simulink model "Ecm_2RC_battery"  (R2022a)
settings: Solver=FixedStepAuto  StartTime=0.0  StopTime=3600  FixedStep=0.1  RelTol=1e-3
values from neighbouring files (symbols this model uses):
  T_init = 293.15    [cell_data.mat]
libraries: fl_lib x1074, LiBatteryElements_lib x540, nesl_utility x102
(part 16 of 18)

== system Ecm_2RC_battery/Subsystem3/Subsystem2/Thermal Model ==
  Battery Thermal Mass : fl_lib/Thermal/Thermal Elements/Thermal Mass  mass=cell_mass kg  sp_heat=cell_Cp_heat J/kg/K  T_specify=on  T_priority=High  T=T_init K  T_nominal_specify=off  T_nominal_unit=K  T_nominal_value=1  Q_specify=off  Q_priority=None  Q=0 W  Q_nominal_specify=off  Q_nominal_unit=W  Q_nominal_value=1
      settings: SourceProductBaseCode=PW,SS,VE
  Controlled Heat Flow Rate Source : fl_lib/Thermal/Thermal Sources/Controlled Heat Flow Rate Source
      settings: SourceProductBaseCode=PW,SS,VE
  Temperature Sensor : fl_lib/Thermal/Thermal Sensors/Temperature Sensor
      settings: SourceProductBaseCode=PW,SS,VE
  Thermal Reference : fl_lib/Thermal/Thermal Elements/Thermal Reference
      settings: SourceProductBaseCode=PW,SS,VE
  Thermal Reference1 : fl_lib/Thermal/Thermal Elements/Thermal Reference
      settings: SourceProductBaseCode=PW,SS,VE
  P_in : PMIOPort  Tag=PMCPort  Side=Left
  H : PMIOPort  Tag=PMCPort  Port=2  Side=Left
  T : PMIOPort  Tag=PMCPort  Port=3  Side=Right
  connections:
  Temperature Sensor/RConn1 -- Thermal Reference1/LConn1
  Temperature Sensor/RConn2 -- T/RConn1
  Controlled Heat Flow Rate Source/RConn2 -- Thermal Reference/LConn1
  Controlled Heat Flow Rate Source/LConn1 -- Temperature Sensor/LConn1 -- Battery Thermal Mass/LConn1 -- H/RConn1
  Controlled Heat Flow Rate Source/RConn1 -- P_in/RConn1

== system Ecm_2RC_battery/Subsystem3/Subsystem3/Sum ==
  Power Sum : fl_lib/Physical Signals/Functions/PS Add
      settings: SourceProductBaseCode=PW,SS,VE
  Power Sum1 : fl_lib/Physical Signals/Functions/PS Add
      settings: SourceProductBaseCode=PW,SS,VE
  I1 : PMIOPort  Side=Right
  I2 : PMIOPort  Port=2  Side=Right
  I3 : PMIOPort  Port=3  Side=Right
  O : PMIOPort  Port=4  Side=Left
  connections:
  Power Sum1/LConn1 -- I2/RConn1
  Power Sum/RConn1 -- O/RConn1
  I3/RConn1 -- Power Sum1/LConn2
  Power Sum1/RConn1 -- Power Sum/LConn2
  I1/RConn1 -- Power Sum/LConn1

== system Ecm_2RC_battery/Subsystem3/Subsystem3/Thermal Model ==
  Battery Thermal Mass : fl_lib/Thermal/Thermal Elements/Thermal Mass  mass=cell_mass kg  sp_heat=cell_Cp_heat J/kg/K  T_specify=on  T_priority=High  T=T_init K  T_nominal_specify=off  T_nominal_unit=K  T_nominal_value=1  Q_specify=off  Q_priority=None  Q=0 W  Q_nominal_specify=off  Q_nominal_unit=W  Q_nominal_value=1
      settings: SourceProductBaseCode=PW,SS,VE
  Controlled Heat Flow Rate Source : fl_lib/Thermal/Thermal Sources/Controlled Heat Flow Rate Source
      settings: SourceProductBaseCode=PW,SS,VE
  Temperature Sensor : fl_lib/Thermal/Thermal Sensors/Temperature Sensor
      settings: SourceProductBaseCode=PW,SS,VE
  Thermal Reference : fl_lib/Thermal/Thermal Elements/Thermal Reference
      settings: SourceProductBaseCode=PW,SS,VE
  Thermal Reference1 : fl_lib/Thermal/Thermal Elements/Thermal Reference
      settings: SourceProductBaseCode=PW,SS,VE
  P_in : PMIOPort  Tag=PMCPort  Side=Left
  H : PMIOPort  Tag=PMCPort  Port=2  Side=Left
  T : PMIOPort  Tag=PMCPort  Port=3  Side=Right
  connections:
  Temperature Sensor/RConn1 -- Thermal Reference1/LConn1
  Temperature Sensor/RConn2 -- T/RConn1
  Controlled Heat Flow Rate Source/RConn2 -- Thermal Reference/LConn1
  Controlled Heat Flow Rate Source/LConn1 -- Temperature Sensor/LConn1 -- Battery Thermal Mass/LConn1 -- H/RConn1
  Controlled Heat Flow Rate Source/RConn1 -- P_in/RConn1

== system Ecm_2RC_battery/Subsystem3/Subsystem4/Sum ==
  Power Sum : fl_lib/Physical Signals/Functions/PS Add
      settings: SourceProductBaseCode=PW,SS,VE
  Power Sum1 : fl_lib/Physical Signals/Functions/PS Add
      settings: SourceProductBaseCode=PW,SS,VE
  I1 : PMIOPort  Side=Right
  I2 : PMIOPort  Port=2  Side=Right
  I3 : PMIOPort  Port=3  Side=Right
  O : PMIOPort  Port=4  Side=Left
  connections:
  Power Sum1/LConn1 -- I2/RConn1
  Power Sum/RConn1 -- O/RConn1
  I3/RConn1 -- Power Sum1/LConn2
  Power Sum1/RConn1 -- Power Sum/LConn2
  I1/RConn1 -- Power Sum/LConn1

== system Ecm_2RC_battery/Subsystem3/Subsystem4/Thermal Model ==
  Battery Thermal Mass : fl_lib/Thermal/Thermal Elements/Thermal Mass  mass=cell_mass kg  sp_heat=cell_Cp_heat J/kg/K  T_specify=on  T_priority=High  T=T_init K  T_nominal_specify=off  T_nominal_unit=K  T_nominal_value=1  Q_specify=off  Q_priority=None  Q=0 W  Q_nominal_specify=off  Q_nominal_unit=W  Q_nominal_value=1
      settings: SourceProductBaseCode=PW,SS,VE
  Controlled Heat Flow Rate Source : fl_lib/Thermal/Thermal Sources/Controlled Heat Flow Rate Source
      settings: SourceProductBaseCode=PW,SS,VE
  Temperature Sensor : fl_lib/Thermal/Thermal Sensors/Temperature Sensor
      settings: SourceProductBaseCode=PW,SS,VE
  Thermal Reference : fl_lib/Thermal/Thermal Elements/Thermal Reference
      settings: SourceProductBaseCode=PW,SS,VE
  Thermal Reference1 : fl_lib/Thermal/Thermal Elements/Thermal Reference
      settings: SourceProductBaseCode=PW,SS,VE
  P_in : PMIOPort  Tag=PMCPort  Side=Left
  H : PMIOPort  Tag=PMCPort  Port=2  Side=Left
  T : PMIOPort  Tag=PMCPort  Port=3  Side=Right
  connections:
  Temperature Sensor/RConn1 -- Thermal Reference1/LConn1
  Temperature Sensor/RConn2 -- T/RConn1
  Controlled Heat Flow Rate Source/RConn2 -- Thermal Reference/LConn1
  Controlled Heat Flow Rate Source/LConn1 -- Temperature Sensor/LConn1 -- Battery Thermal Mass/LConn1 -- H/RConn1
  Controlled Heat Flow Rate Source/RConn1 -- P_in/RConn1

== system Ecm_2RC_battery/Subsystem3/Subsystem5/Sum ==
  Power Sum : fl_lib/Physical Signals/Functions/PS Add
      settings: SourceProductBaseCode=PW,SS,VE
  Power Sum1 : fl_lib/Physical Signals/Functions/PS Add
      settings: SourceProductBaseCode=PW,SS,VE
  I1 : PMIOPort  Side=Right
  I2 : PMIOPort  Port=2  Side=Right
  I3 : PMIOPort  Port=3  Side=Right
  O : PMIOPort  Port=4  Side=Left
  connections:
  Power Sum1/LConn1 -- I2/RConn1
  Power Sum/RConn1 -- O/RConn1
  I3/RConn1 -- Power Sum1/LConn2
  Power Sum1/RConn1 -- Power Sum/LConn2
  I1/RConn1 -- Power Sum/LConn1

== system Ecm_2RC_battery/Subsystem3/Subsystem5/Thermal Model ==
  Battery Thermal Mass : fl_lib/Thermal/Thermal Elements/Thermal Mass  mass=cell_mass kg  sp_heat=cell_Cp_heat J/kg/K  T_specify=on  T_priority=High  T=T_init K  T_nominal_specify=off  T_nominal_unit=K  T_nominal_value=1  Q_specify=off  Q_priority=None  Q=0 W  Q_nominal_specify=off  Q_nominal_unit=W  Q_nominal_value=1
      settings: SourceProductBaseCode=PW,SS,VE
  Controlled Heat Flow Rate Source : fl_lib/Thermal/Thermal Sources/Controlled Heat Flow Rate Source
      settings: SourceProductBaseCode=PW,SS,VE
  Temperature Sensor : fl_lib/Thermal/Thermal Sensors/Temperature Sensor
      settings: SourceProductBaseCode=PW,SS,VE
  Thermal Reference : fl_lib/Thermal/Thermal Elements/Thermal Reference
      settings: SourceProductBaseCode=PW,SS,VE
  Thermal Reference1 : fl_lib/Thermal/Thermal Elements/Thermal Reference
      settings: SourceProductBaseCode=PW,SS,VE
  P_in : PMIOPort  Tag=PMCPort  Side=Left
  H : PMIOPort  Tag=PMCPort  Port=2  Side=Left
  T : PMIOPort  Tag=PMCPort  Port=3  Side=Right
  connections:
  Temperature Sensor/RConn1 -- Thermal Reference1/LConn1
  Temperature Sensor/RConn2 -- T/RConn1
  Controlled Heat Flow Rate Source/RConn2 -- Thermal Reference/LConn1
  Controlled Heat Flow Rate Source/LConn1 -- Temperature Sensor/LConn1 -- Battery Thermal Mass/LConn1 -- H/RConn1
  Controlled Heat Flow Rate Source/RConn1 -- P_in/RConn1

== system Ecm_2RC_battery/Subsystem3/Subsystem6/Sum ==
  Power Sum : fl_lib/Physical Signals/Functions/PS Add
      settings: SourceProductBaseCode=PW,SS,VE
  Power Sum1 : fl_lib/Physical Signals/Functions/PS Add
      settings: SourceProductBaseCode=PW,SS,VE
  I1 : PMIOPort  Side=Right
  I2 : PMIOPort  Port=2  Side=Right
  I3 : PMIOPort  Port=3  Side=Right
  O : PMIOPort  Port=4  Side=Left
  connections:
  Power Sum1/LConn1 -- I2/RConn1
  Power Sum/RConn1 -- O/RConn1
  I3/RConn1 -- Power Sum1/LConn2
  Power Sum1/RConn1 -- Power Sum/LConn2
  I1/RConn1 -- Power Sum/LConn1

== system Ecm_2RC_battery/Subsystem3/Subsystem6/Thermal Model ==
  Battery Thermal Mass : fl_lib/Thermal/Thermal Elements/Thermal Mass  mass=cell_mass kg  sp_heat=cell_Cp_heat J/kg/K  T_specify=on  T_priority=High  T=T_init K  T_nominal_specify=off  T_nominal_unit=K  T_nominal_value=1  Q_specify=off  Q_priority=None  Q=0 W  Q_nominal_specify=off  Q_nominal_unit=W  Q_nominal_value=1
      settings: SourceProductBaseCode=PW,SS,VE
  Controlled Heat Flow Rate Source : fl_lib/Thermal/Thermal Sources/Controlled Heat Flow Rate Source
      settings: SourceProductBaseCode=PW,SS,VE
  Temperature Sensor : fl_lib/Thermal/Thermal Sensors/Temperature Sensor
      settings: SourceProductBaseCode=PW,SS,VE
  Thermal Reference : fl_lib/Thermal/Thermal Elements/Thermal Reference
      settings: SourceProductBaseCode=PW,SS,VE
  Thermal Reference1 : fl_lib/Thermal/Thermal Elements/Thermal Reference
      settings: SourceProductBaseCode=PW,SS,VE
  P_in : PMIOPort  Tag=PMCPort  Side=Left
  H : PMIOPort  Tag=PMCPort  Port=2  Side=Left
  T : PMIOPort  Tag=PMCPort  Port=3  Side=Right
  connections:
  Temperature Sensor/RConn1 -- Thermal Reference1/LConn1
  Temperature Sensor/RConn2 -- T/RConn1
  Controlled Heat Flow Rate Source/RConn2 -- Thermal Reference/LConn1
  Controlled Heat Flow Rate Source/LConn1 -- Temperature Sensor/LConn1 -- Battery Thermal Mass/LConn1 -- H/RConn1
  Controlled Heat Flow Rate Source/RConn1 -- P_in/RConn1

== system Ecm_2RC_battery/Subsystem3/Subsystem7/Sum ==
  Power Sum : fl_lib/Physical Signals/Functions/PS Add
      settings: SourceProductBaseCode=PW,SS,VE
  Power Sum1 : fl_lib/Physical Signals/Functions/PS Add
      settings: SourceProductBaseCode=PW,SS,VE
  I1 : PMIOPort  Side=Right
  I2 : PMIOPort  Port=2  Side=Right
  I3 : PMIOPort  Port=3  Side=Right
  O : PMIOPort  Port=4  Side=Left
  connections:
  Power Sum1/LConn1 -- I2/RConn1
  Power Sum/RConn1 -- O/RConn1
  I3/RConn1 -- Power Sum1/LConn2
  Power Sum1/RConn1 -- Power Sum/LConn2
  I1/RConn1 -- Power Sum/LConn1

== system Ecm_2RC_battery/Subsystem3/Subsystem7/Thermal Model ==
  Battery Thermal Mass : fl_lib/Thermal/Thermal Elements/Thermal Mass  mass=cell_mass kg  sp_heat=cell_Cp_heat J/kg/K  T_specify=on  T_priority=High  T=T_init K  T_nominal_specify=off  T_nominal_unit=K  T_nominal_value=1  Q_specify=off  Q_priority=None  Q=0 W  Q_nominal_specify=off  Q_nominal_unit=W  Q_nominal_value=1
      settings: SourceProductBaseCode=PW,SS,VE
  Controlled Heat Flow Rate Source : fl_lib/Thermal/Thermal Sources/Controlled Heat Flow Rate Source
      settings: SourceProductBaseCode=PW,SS,VE
  Temperature Sensor : fl_lib/Thermal/Thermal Sensors/Temperature Sensor
      settings: SourceProductBaseCode=PW,SS,VE
  Thermal Reference : fl_lib/Thermal/Thermal Elements/Thermal Reference
      settings: SourceProductBaseCode=PW,SS,VE
  Thermal Reference1 : fl_lib/Thermal/Thermal Elements/Thermal Reference
      settings: SourceProductBaseCode=PW,SS,VE
  P_in : PMIOPort  Tag=PMCPort  Side=Left
  H : PMIOPort  Tag=PMCPort  Port=2  Side=Left
  T : PMIOPort  Tag=PMCPort  Port=3  Side=Right
  connections:
  Temperature Sensor/RConn1 -- Thermal Reference1/LConn1
  Temperature Sensor/RConn2 -- T/RConn1
  Controlled Heat Flow Rate Source/RConn2 -- Thermal Reference/LConn1
  Controlled Heat Flow Rate Source/LConn1 -- Temperature Sensor/LConn1 -- Battery Thermal Mass/LConn1 -- H/RConn1
  Controlled Heat Flow Rate Source/RConn1 -- P_in/RConn1

== system Ecm_2RC_battery/Subsystem3/Subsystem8/Sum ==
  Power Sum : fl_lib/Physical Signals/Functions/PS Add
      settings: SourceProductBaseCode=PW,SS,VE
  Power Sum1 : fl_lib/Physical Signals/Functions/PS Add
      settings: SourceProductBaseCode=PW,SS,VE
  I1 : PMIOPort  Side=Right
  I2 : PMIOPort  Port=2  Side=Right
  I3 : PMIOPort  Port=3  Side=Right
  O : PMIOPort  Port=4  Side=Left
  connections:
  Power Sum1/LConn1 -- I2/RConn1
  Power Sum/RConn1 -- O/RConn1
  I3/RConn1 -- Power Sum1/LConn2
  Power Sum1/RConn1 -- Power Sum/LConn2
  I1/RConn1 -- Power Sum/LConn1

== system Ecm_2RC_battery/Subsystem3/Subsystem8/Thermal Model ==
  Battery Thermal Mass : fl_lib/Thermal/Thermal Elements/Thermal Mass  mass=cell_mass kg  sp_heat=cell_Cp_heat J/kg/K  T_specify=on  T_priority=High  T=T_init K  T_nominal_specify=off  T_nominal_unit=K  T_nominal_value=1  Q_specify=off  Q_priority=None  Q=0 W  Q_nominal_specify=off  Q_nominal_unit=W  Q_nominal_value=1
      settings: SourceProductBaseCode=PW,SS,VE
  Controlled Heat Flow Rate Source : fl_lib/Thermal/Thermal Sources/Controlled Heat Flow Rate Source
      settings: SourceProductBaseCode=PW,SS,VE
  Temperature Sensor : fl_lib/Thermal/Thermal Sensors/Temperature Sensor
      settings: SourceProductBaseCode=PW,SS,VE
  Thermal Reference : fl_lib/Thermal/Thermal Elements/Thermal Reference
      settings: SourceProductBaseCode=PW,SS,VE
  Thermal Reference1 : fl_lib/Thermal/Thermal Elements/Thermal Reference
      settings: SourceProductBaseCode=PW,SS,VE
  P_in : PMIOPort  Tag=PMCPort  Side=Left
  H : PMIOPort  Tag=PMCPort  Port=2  Side=Left
  T : PMIOPort  Tag=PMCPort  Port=3  Side=Right
  connections:
  Temperature Sensor/RConn1 -- Thermal Reference1/LConn1
  Temperature Sensor/RConn2 -- T/RConn1
  Controlled Heat Flow Rate Source/RConn2 -- Thermal Reference/LConn1
  Controlled Heat Flow Rate Source/LConn1 -- Temperature Sensor/LConn1 -- Battery Thermal Mass/LConn1 -- H/RConn1
  Controlled Heat Flow Rate Source/RConn1 -- P_in/RConn1

== system Ecm_2RC_battery/Subsystem3/Subsystem9/Sum ==
  Power Sum : fl_lib/Physical Signals/Functions/PS Add
      settings: SourceProductBaseCode=PW,SS,VE
  Power Sum1 : fl_lib/Physical Signals/Functions/PS Add
      settings: SourceProductBaseCode=PW,SS,VE
  I1 : PMIOPort  Side=Right
  I2 : PMIOPort  Port=2  Side=Right
  I3 : PMIOPort  Port=3  Side=Right
  O : PMIOPort  Port=4  Side=Left
  connections:
  Power Sum1/LConn1 -- I2/RConn1
  Power Sum/RConn1 -- O/RConn1
  I3/RConn1 -- Power Sum1/LConn2
  Power Sum1/RConn1 -- Power Sum/LConn2
  I1/RConn1 -- Power Sum/LConn1

== system Ecm_2RC_battery/Subsystem3/Subsystem9/Thermal Model ==
  Battery Thermal Mass : fl_lib/Thermal/Thermal Elements/Thermal Mass  mass=cell_mass kg  sp_heat=cell_Cp_heat J/kg/K  T_specify=on  T_priority=High  T=T_init K  T_nominal_specify=off  T_nominal_unit=K  T_nominal_value=1  Q_specify=off  Q_priority=None  Q=0 W  Q_nominal_specify=off  Q_nominal_unit=W  Q_nominal_value=1
      settings: SourceProductBaseCode=PW,SS,VE
  Controlled Heat Flow Rate Source : fl_lib/Thermal/Thermal Sources/Controlled Heat Flow Rate Source
      settings: SourceProductBaseCode=PW,SS,VE
  Temperature Sensor : fl_lib/Thermal/Thermal Sensors/Temperature Sensor
      settings: SourceProductBaseCode=PW,SS,VE
  Thermal Reference : fl_lib/Thermal/Thermal Elements/Thermal Reference
      settings: SourceProductBaseCode=PW,SS,VE
  Thermal Reference1 : fl_lib/Thermal/Thermal Elements/Thermal Reference
      settings: SourceProductBaseCode=PW,SS,VE
  P_in : PMIOPort  Tag=PMCPort  Side=Left
  H : PMIOPort  Tag=PMCPort  Port=2  Side=Left
  T : PMIOPort  Tag=PMCPort  Port=3  Side=Right
  connections:
  Temperature Sensor/RConn1 -- Thermal Reference1/LConn1
  Temperature Sensor/RConn2 -- T/RConn1
  Controlled Heat Flow Rate Source/RConn2 -- Thermal Reference/LConn1
  Controlled Heat Flow Rate Source/LConn1 -- Temperature Sensor/LConn1 -- Battery Thermal Mass/LConn1 -- H/RConn1
  Controlled Heat Flow Rate Source/RConn1 -- P_in/RConn1

== system Ecm_2RC_battery/Subsystem4/Subsystem/Sum ==
  Power Sum : fl_lib/Physical Signals/Functions/PS Add
      settings: SourceProductBaseCode=PW,SS,VE
  Power Sum1 : fl_lib/Physical Signals/Functions/PS Add
      settings: SourceProductBaseCode=PW,SS,VE
  I1 : PMIOPort  Side=Right
  I2 : PMIOPort  Port=2  Side=Right
  I3 : PMIOPort  Port=3  Side=Right
  O : PMIOPort  Port=4  Side=Left
  connections:
  Power Sum1/LConn1 -- I2/RConn1
  Power Sum/RConn1 -- O/RConn1
  I3/RConn1 -- Power Sum1/LConn2
  Power Sum1/RConn1 -- Power Sum/LConn2
  I1/RConn1 -- Power Sum/LConn1

== system Ecm_2RC_battery/Subsystem4/Subsystem/Thermal Model ==
  Battery Thermal Mass : fl_lib/Thermal/Thermal Elements/Thermal Mass  mass=cell_mass kg  sp_heat=cell_Cp_heat J/kg/K  T_specify=on  T_priority=High  T=T_init K  T_nominal_specify=off  T_nominal_unit=K  T_nominal_value=1  Q_specify=off  Q_priority=None  Q=0 W  Q_nominal_specify=off  Q_nominal_unit=W  Q_nominal_value=1
      settings: SourceProductBaseCode=PW,SS,VE
  Controlled Heat Flow Rate Source : fl_lib/Thermal/Thermal Sources/Controlled Heat Flow Rate Source
      settings: SourceProductBaseCode=PW,SS,VE
  Temperature Sensor : fl_lib/Thermal/Thermal Sensors/Temperature Sensor
      settings: SourceProductBaseCode=PW,SS,VE
  Thermal Reference : fl_lib/Thermal/Thermal Elements/Thermal Reference
      settings: SourceProductBaseCode=PW,SS,VE
  Thermal Reference1 : fl_lib/Thermal/Thermal Elements/Thermal Reference
      settings: SourceProductBaseCode=PW,SS,VE
  P_in : PMIOPort  Tag=PMCPort  Side=Left
  H : PMIOPort  Tag=PMCPort  Port=2  Side=Left
  T : PMIOPort  Tag=PMCPort  Port=3  Side=Right
  connections:
  Temperature Sensor/RConn1 -- Thermal Reference1/LConn1
  Temperature Sensor/RConn2 -- T/RConn1
  Controlled Heat Flow Rate Source/RConn2 -- Thermal Reference/LConn1
  Controlled Heat Flow Rate Source/LConn1 -- Temperature Sensor/LConn1 -- Battery Thermal Mass/LConn1 -- H/RConn1
  Controlled Heat Flow Rate Source/RConn1 -- P_in/RConn1

== system Ecm_2RC_battery/Subsystem4/Subsystem1/Sum ==
  Power Sum : fl_lib/Physical Signals/Functions/PS Add
      settings: SourceProductBaseCode=PW,SS,VE
  Power Sum1 : fl_lib/Physical Signals/Functions/PS Add
      settings: SourceProductBaseCode=PW,SS,VE
  I1 : PMIOPort  Side=Right
  I2 : PMIOPort  Port=2  Side=Right
  I3 : PMIOPort  Port=3  Side=Right
  O : PMIOPort  Port=4  Side=Left
  connections:
  Power Sum1/LConn1 -- I2/RConn1
  Power Sum/RConn1 -- O/RConn1
  I3/RConn1 -- Power Sum1/LConn2
  Power Sum1/RConn1 -- Power Sum/LConn2
  I1/RConn1 -- Power Sum/LConn1

== system Ecm_2RC_battery/Subsystem4/Subsystem1/Thermal Model ==
  Battery Thermal Mass : fl_lib/Thermal/Thermal Elements/Thermal Mass  mass=cell_mass kg  sp_heat=cell_Cp_heat J/kg/K  T_specify=on  T_priority=High  T=T_init K  T_nominal_specify=off  T_nominal_unit=K  T_nominal_value=1  Q_specify=off  Q_priority=None  Q=0 W  Q_nominal_specify=off  Q_nominal_unit=W  Q_nominal_value=1
      settings: SourceProductBaseCode=PW,SS,VE
  Controlled Heat Flow Rate Source : fl_lib/Thermal/Thermal Sources/Controlled Heat Flow Rate Source
      settings: SourceProductBaseCode=PW,SS,VE
  Temperature Sensor : fl_lib/Thermal/Thermal Sensors/Temperature Sensor
      settings: SourceProductBaseCode=PW,SS,VE
  Thermal Reference : fl_lib/Thermal/Thermal Elements/Thermal Reference
      settings: SourceProductBaseCode=PW,SS,VE
  Thermal Reference1 : fl_lib/Thermal/Thermal Elements/Thermal Reference
      settings: SourceProductBaseCode=PW,SS,VE
  P_in : PMIOPort  Tag=PMCPort  Side=Left
  H : PMIOPort  Tag=PMCPort  Port=2  Side=Left
  T : PMIOPort  Tag=PMCPort  Port=3  Side=Right
  connections:
  Temperature Sensor/RConn1 -- Thermal Reference1/LConn1
  Temperature Sensor/RConn2 -- T/RConn1
  Controlled Heat Flow Rate Source/RConn2 -- Thermal Reference/LConn1
  Controlled Heat Flow Rate Source/LConn1 -- Temperature Sensor/LConn1 -- Battery Thermal Mass/LConn1 -- H/RConn1
  Controlled Heat Flow Rate Source/RConn1 -- P_in/RConn1

== system Ecm_2RC_battery/Subsystem4/Subsystem2/Sum ==
  Power Sum : fl_lib/Physical Signals/Functions/PS Add
      settings: SourceProductBaseCode=PW,SS,VE
  Power Sum1 : fl_lib/Physical Signals/Functions/PS Add
      settings: SourceProductBaseCode=PW,SS,VE
  I1 : PMIOPort  Side=Right
  I2 : PMIOPort  Port=2  Side=Right
  I3 : PMIOPort  Port=3  Side=Right
  O : PMIOPort  Port=4  Side=Left
  connections:
  Power Sum1/LConn1 -- I2/RConn1
  Power Sum/RConn1 -- O/RConn1
  I3/RConn1 -- Power Sum1/LConn2
  Power Sum1/RConn1 -- Power Sum/LConn2
  I1/RConn1 -- Power Sum/LConn1

== system Ecm_2RC_battery/Subsystem4/Subsystem2/Thermal Model ==
  Battery Thermal Mass : fl_lib/Thermal/Thermal Elements/Thermal Mass  mass=cell_mass kg  sp_heat=cell_Cp_heat J/kg/K  T_specify=on  T_priority=High  T=T_init K  T_nominal_specify=off  T_nominal_unit=K  T_nominal_value=1  Q_specify=off  Q_priority=None  Q=0 W  Q_nominal_specify=off  Q_nominal_unit=W  Q_nominal_value=1
      settings: SourceProductBaseCode=PW,SS,VE
  Controlled Heat Flow Rate Source : fl_lib/Thermal/Thermal Sources/Controlled Heat Flow Rate Source
      settings: SourceProductBaseCode=PW,SS,VE
  Temperature Sensor : fl_lib/Thermal/Thermal Sensors/Temperature Sensor
      settings: SourceProductBaseCode=PW,SS,VE
  Thermal Reference : fl_lib/Thermal/Thermal Elements/Thermal Reference
      settings: SourceProductBaseCode=PW,SS,VE
  Thermal Reference1 : fl_lib/Thermal/Thermal Elements/Thermal Reference
      settings: SourceProductBaseCode=PW,SS,VE
  P_in : PMIOPort  Tag=PMCPort  Side=Left
  H : PMIOPort  Tag=PMCPort  Port=2  Side=Left
  T : PMIOPort  Tag=PMCPort  Port=3  Side=Right
  connections:
  Temperature Sensor/RConn1 -- Thermal Reference1/LConn1
  Temperature Sensor/RConn2 -- T/RConn1
  Controlled Heat Flow Rate Source/RConn2 -- Thermal Reference/LConn1
  Controlled Heat Flow Rate Source/LConn1 -- Temperature Sensor/LConn1 -- Battery Thermal Mass/LConn1 -- H/RConn1
  Controlled Heat Flow Rate Source/RConn1 -- P_in/RConn1

== system Ecm_2RC_battery/Subsystem4/Subsystem3/Sum ==
  Power Sum : fl_lib/Physical Signals/Functions/PS Add
      settings: SourceProductBaseCode=PW,SS,VE
  Power Sum1 : fl_lib/Physical Signals/Functions/PS Add
      settings: SourceProductBaseCode=PW,SS,VE
  I1 : PMIOPort  Side=Right
  I2 : PMIOPort  Port=2  Side=Right
  I3 : PMIOPort  Port=3  Side=Right
  O : PMIOPort  Port=4  Side=Left
  connections:
  Power Sum1/LConn1 -- I2/RConn1
  Power Sum/RConn1 -- O/RConn1
  I3/RConn1 -- Power Sum1/LConn2
  Power Sum1/RConn1 -- Power Sum/LConn2
  I1/RConn1 -- Power Sum/LConn1

== system Ecm_2RC_battery/Subsystem4/Subsystem3/Thermal Model ==
  Battery Thermal Mass : fl_lib/Thermal/Thermal Elements/Thermal Mass  mass=cell_mass kg  sp_heat=cell_Cp_heat J/kg/K  T_specify=on  T_priority=High  T=T_init K  T_nominal_specify=off  T_nominal_unit=K  T_nominal_value=1  Q_specify=off  Q_priority=None  Q=0 W  Q_nominal_specify=off  Q_nominal_unit=W  Q_nominal_value=1
      settings: SourceProductBaseCode=PW,SS,VE
  Controlled Heat Flow Rate Source : fl_lib/Thermal/Thermal Sources/Controlled Heat Flow Rate Source
      settings: SourceProductBaseCode=PW,SS,VE
  Temperature Sensor : fl_lib/Thermal/Thermal Sensors/Temperature Sensor
      settings: SourceProductBaseCode=PW,SS,VE
  Thermal Reference : fl_lib/Thermal/Thermal Elements/Thermal Reference
      settings: SourceProductBaseCode=PW,SS,VE
  Thermal Reference1 : fl_lib/Thermal/Thermal Elements/Thermal Reference
      settings: SourceProductBaseCode=PW,SS,VE
  P_in : PMIOPort  Tag=PMCPort  Side=Left
  H : PMIOPort  Tag=PMCPort  Port=2  Side=Left
  T : PMIOPort  Tag=PMCPort  Port=3  Side=Right
  connections:
  Temperature Sensor/RConn1 -- Thermal Reference1/LConn1
  Temperature Sensor/RConn2 -- T/RConn1
  Controlled Heat Flow Rate Source/RConn2 -- Thermal Reference/LConn1
  Controlled Heat Flow Rate Source/LConn1 -- Temperature Sensor/LConn1 -- Battery Thermal Mass/LConn1 -- H/RConn1
  Controlled Heat Flow Rate Source/RConn1 -- P_in/RConn1

== system Ecm_2RC_battery/Subsystem4/Subsystem4/Sum ==
  Power Sum : fl_lib/Physical Signals/Functions/PS Add
      settings: SourceProductBaseCode=PW,SS,VE
  Power Sum1 : fl_lib/Physical Signals/Functions/PS Add
      settings: SourceProductBaseCode=PW,SS,VE
  I1 : PMIOPort  Side=Right
  I2 : PMIOPort  Port=2  Side=Right
  I3 : PMIOPort  Port=3  Side=Right
  O : PMIOPort  Port=4  Side=Left
  connections:
  Power Sum1/LConn1 -- I2/RConn1
  Power Sum/RConn1 -- O/RConn1
  I3/RConn1 -- Power Sum1/LConn2
  Power Sum1/RConn1 -- Power Sum/LConn2
  I1/RConn1 -- Power Sum/LConn1

== system Ecm_2RC_battery/Subsystem4/Subsystem4/Thermal Model ==
  Battery Thermal Mass : fl_lib/Thermal/Thermal Elements/Thermal Mass  mass=cell_mass kg  sp_heat=cell_Cp_heat J/kg/K  T_specify=on  T_priority=High  T=T_init K  T_nominal_specify=off  T_nominal_unit=K  T_nominal_value=1  Q_specify=off  Q_priority=None  Q=0 W  Q_nominal_specify=off  Q_nominal_unit=W  Q_nominal_value=1
      settings: SourceProductBaseCode=PW,SS,VE
  Controlled Heat Flow Rate Source : fl_lib/Thermal/Thermal Sources/Controlled Heat Flow Rate Source
      settings: SourceProductBaseCode=PW,SS,VE
  Temperature Sensor : fl_lib/Thermal/Thermal Sensors/Temperature Sensor
      settings: SourceProductBaseCode=PW,SS,VE
  Thermal Reference : fl_lib/Thermal/Thermal Elements/Thermal Reference
      settings: SourceProductBaseCode=PW,SS,VE
  Thermal Reference1 : fl_lib/Thermal/Thermal Elements/Thermal Reference
      settings: SourceProductBaseCode=PW,SS,VE
  P_in : PMIOPort  Tag=PMCPort  Side=Left
  H : PMIOPort  Tag=PMCPort  Port=2  Side=Left
  T : PMIOPort  Tag=PMCPort  Port=3  Side=Right
  connections:
  Temperature Sensor/RConn1 -- Thermal Reference1/LConn1
  Temperature Sensor/RConn2 -- T/RConn1
  Controlled Heat Flow Rate Source/RConn2 -- Thermal Reference/LConn1
  Controlled Heat Flow Rate Source/LConn1 -- Temperature Sensor/LConn1 -- Battery Thermal Mass/LConn1 -- H/RConn1
  Controlled Heat Flow Rate Source/RConn1 -- P_in/RConn1

== system Ecm_2RC_battery/Subsystem4/Subsystem5/Sum ==
  Power Sum : fl_lib/Physical Signals/Functions/PS Add
      settings: SourceProductBaseCode=PW,SS,VE
  Power Sum1 : fl_lib/Physical Signals/Functions/PS Add
      settings: SourceProductBaseCode=PW,SS,VE
  I1 : PMIOPort  Side=Right
  I2 : PMIOPort  Port=2  Side=Right
  I3 : PMIOPort  Port=3  Side=Right
  O : PMIOPort  Port=4  Side=Left
  connections:
  Power Sum1/LConn1 -- I2/RConn1
  Power Sum/RConn1 -- O/RConn1
  I3/RConn1 -- Power Sum1/LConn2
  Power Sum1/RConn1 -- Power Sum/LConn2
  I1/RConn1 -- Power Sum/LConn1

== system Ecm_2RC_battery/Subsystem4/Subsystem5/Thermal Model ==
  Battery Thermal Mass : fl_lib/Thermal/Thermal Elements/Thermal Mass  mass=cell_mass kg  sp_heat=cell_Cp_heat J/kg/K  T_specify=on  T_priority=High  T=T_init K  T_nominal_specify=off  T_nominal_unit=K  T_nominal_value=1  Q_specify=off  Q_priority=None  Q=0 W  Q_nominal_specify=off  Q_nominal_unit=W  Q_nominal_value=1
      settings: SourceProductBaseCode=PW,SS,VE
  Controlled Heat Flow Rate Source : fl_lib/Thermal/Thermal Sources/Controlled Heat Flow Rate Source
      settings: SourceProductBaseCode=PW,SS,VE
  Temperature Sensor : fl_lib/Thermal/Thermal Sensors/Temperature Sensor
      settings: SourceProductBaseCode=PW,SS,VE
  Thermal Reference : fl_lib/Thermal/Thermal Elements/Thermal Reference
      settings: SourceProductBaseCode=PW,SS,VE
  Thermal Reference1 : fl_lib/Thermal/Thermal Elements/Thermal Reference
      settings: SourceProductBaseCode=PW,SS,VE
  P_in : PMIOPort  Tag=PMCPort  Side=Left
  H : PMIOPort  Tag=PMCPort  Port=2  Side=Left
  T : PMIOPort  Tag=PMCPort  Port=3  Side=Right
  connections:
  Temperature Sensor/RConn1 -- Thermal Reference1/LConn1
  Temperature Sensor/RConn2 -- T/RConn1
  Controlled Heat Flow Rate Source/RConn2 -- Thermal Reference/LConn1
  Controlled Heat Flow Rate Source/LConn1 -- Temperature Sensor/LConn1 -- Battery Thermal Mass/LConn1 -- H/RConn1
  Controlled Heat Flow Rate Source/RConn1 -- P_in/RConn1

== system Ecm_2RC_battery/Subsystem4/Subsystem6/Sum ==
  Power Sum : fl_lib/Physical Signals/Functions/PS Add
      settings: SourceProductBaseCode=PW,SS,VE
  Power Sum1 : fl_lib/Physical Signals/Functions/PS Add
      settings: SourceProductBaseCode=PW,SS,VE
  I1 : PMIOPort  Side=Right
  I2 : PMIOPort  Port=2  Side=Right
  I3 : PMIOPort  Port=3  Side=Right
  O : PMIOPort  Port=4  Side=Left
  connections:
  Power Sum1/LConn1 -- I2/RConn1
  Power Sum/RConn1 -- O/RConn1
  I3/RConn1 -- Power Sum1/LConn2
  Power Sum1/RConn1 -- Power Sum/LConn2
  I1/RConn1 -- Power Sum/LConn1

== system Ecm_2RC_battery/Subsystem4/Subsystem6/Thermal Model ==
  Battery Thermal Mass : fl_lib/Thermal/Thermal Elements/Thermal Mass  mass=cell_mass kg  sp_heat=cell_Cp_heat J/kg/K  T_specify=on  T_priority=High  T=T_init K  T_nominal_specify=off  T_nominal_unit=K  T_nominal_value=1  Q_specify=off  Q_priority=None  Q=0 W  Q_nominal_specify=off  Q_nominal_unit=W  Q_nominal_value=1
      settings: SourceProductBaseCode=PW,SS,VE
  Controlled Heat Flow Rate Source : fl_lib/Thermal/Thermal Sources/Controlled Heat Flow Rate Source
      settings: SourceProductBaseCode=PW,SS,VE
  Temperature Sensor : fl_lib/Thermal/Thermal Sensors/Temperature Sensor
      settings: SourceProductBaseCode=PW,SS,VE
  Thermal Reference : fl_lib/Thermal/Thermal Elements/Thermal Reference
      settings: SourceProductBaseCode=PW,SS,VE
  Thermal Reference1 : fl_lib/Thermal/Thermal Elements/Thermal Reference
      settings: SourceProductBaseCode=PW,SS,VE
  P_in : PMIOPort  Tag=PMCPort  Side=Left
  H : PMIOPort  Tag=PMCPort  Port=2  Side=Left
  T : PMIOPort  Tag=PMCPort  Port=3  Side=Right
  connections:
  Temperature Sensor/RConn1 -- Thermal Reference1/LConn1
  Temperature Sensor/RConn2 -- T/RConn1
  Controlled Heat Flow Rate Source/RConn2 -- Thermal Reference/LConn1
  Controlled Heat Flow Rate Source/LConn1 -- Temperature Sensor/LConn1 -- Battery Thermal Mass/LConn1 -- H/RConn1
  Controlled Heat Flow Rate Source/RConn1 -- P_in/RConn1

== system Ecm_2RC_battery/Subsystem4/Subsystem7/Sum ==
  Power Sum : fl_lib/Physical Signals/Functions/PS Add
      settings: SourceProductBaseCode=PW,SS,VE
  Power Sum1 : fl_lib/Physical Signals/Functions/PS Add
      settings: SourceProductBaseCode=PW,SS,VE
  I1 : PMIOPort  Side=Right
  I2 : PMIOPort  Port=2  Side=Right
  I3 : PMIOPort  Port=3  Side=Right
  O : PMIOPort  Port=4  Side=Left
  connections:
  Power Sum1/LConn1 -- I2/RConn1
  Power Sum/RConn1 -- O/RConn1
  I3/RConn1 -- Power Sum1/LConn2
  Power Sum1/RConn1 -- Power Sum/LConn2
  I1/RConn1 -- Power Sum/LConn1

== system Ecm_2RC_battery/Subsystem4/Subsystem7/Thermal Model ==
  Battery Thermal Mass : fl_lib/Thermal/Thermal Elements/Thermal Mass  mass=cell_mass kg  sp_heat=cell_Cp_heat J/kg/K  T_specify=on  T_priority=High  T=T_init K  T_nominal_specify=off  T_nominal_unit=K  T_nominal_value=1  Q_specify=off  Q_priority=None  Q=0 W  Q_nominal_specify=off  Q_nominal_unit=W  Q_nominal_value=1
      settings: SourceProductBaseCode=PW,SS,VE
  Controlled Heat Flow Rate Source : fl_lib/Thermal/Thermal Sources/Controlled Heat Flow Rate Source
      settings: SourceProductBaseCode=PW,SS,VE
  Temperature Sensor : fl_lib/Thermal/Thermal Sensors/Temperature Sensor
      settings: SourceProductBaseCode=PW,SS,VE
  Thermal Reference : fl_lib/Thermal/Thermal Elements/Thermal Reference
      settings: SourceProductBaseCode=PW,SS,VE
  Thermal Reference1 : fl_lib/Thermal/Thermal Elements/Thermal Reference
      settings: SourceProductBaseCode=PW,SS,VE
  P_in : PMIOPort  Tag=PMCPort  Side=Left
  H : PMIOPort  Tag=PMCPort  Port=2  Side=Left
  T : PMIOPort  Tag=PMCPort  Port=3  Side=Right
  connections:
  Temperature Sensor/RConn1 -- Thermal Reference1/LConn1
  Temperature Sensor/RConn2 -- T/RConn1
  Controlled Heat Flow Rate Source/RConn2 -- Thermal Reference/LConn1
  Controlled Heat Flow Rate Source/LConn1 -- Temperature Sensor/LConn1 -- Battery Thermal Mass/LConn1 -- H/RConn1
  Controlled Heat Flow Rate Source/RConn1 -- P_in/RConn1

== system Ecm_2RC_battery/Subsystem4/Subsystem8/Sum ==
  Power Sum : fl_lib/Physical Signals/Functions/PS Add
      settings: SourceProductBaseCode=PW,SS,VE
  Power Sum1 : fl_lib/Physical Signals/Functions/PS Add
      settings: SourceProductBaseCode=PW,SS,VE
  I1 : PMIOPort  Side=Right
  I2 : PMIOPort  Port=2  Side=Right
  I3 : PMIOPort  Port=3  Side=Right
  O : PMIOPort  Port=4  Side=Left
  connections:
  Power Sum1/LConn1 -- I2/RConn1
  Power Sum/RConn1 -- O/RConn1
  I3/RConn1 -- Power Sum1/LConn2
  Power Sum1/RConn1 -- Power Sum/LConn2
  I1/RConn1 -- Power Sum/LConn1

== system Ecm_2RC_battery/Subsystem4/Subsystem8/Thermal Model ==
  Battery Thermal Mass : fl_lib/Thermal/Thermal Elements/Thermal Mass  mass=cell_mass kg  sp_heat=cell_Cp_heat J/kg/K  T_specify=on  T_priority=High  T=T_init K  T_nominal_specify=off  T_nominal_unit=K  T_nominal_value=1  Q_specify=off  Q_priority=None  Q=0 W  Q_nominal_specify=off  Q_nominal_unit=W  Q_nominal_value=1
      settings: SourceProductBaseCode=PW,SS,VE
  Controlled Heat Flow Rate Source : fl_lib/Thermal/Thermal Sources/Controlled Heat Flow Rate Source
      settings: SourceProductBaseCode=PW,SS,VE
  Temperature Sensor : fl_lib/Thermal/Thermal Sensors/Temperature Sensor
      settings: SourceProductBaseCode=PW,SS,VE
  Thermal Reference : fl_lib/Thermal/Thermal Elements/Thermal Reference
      settings: SourceProductBaseCode=PW,SS,VE
  Thermal Reference1 : fl_lib/Thermal/Thermal Elements/Thermal Reference
      settings: SourceProductBaseCode=PW,SS,VE
  P_in : PMIOPort  Tag=PMCPort  Side=Left
  H : PMIOPort  Tag=PMCPort  Port=2  Side=Left
  T : PMIOPort  Tag=PMCPort  Port=3  Side=Right
  connections:
  Temperature Sensor/RConn1 -- Thermal Reference1/LConn1
  Temperature Sensor/RConn2 -- T/RConn1
  Controlled Heat Flow Rate Source/RConn2 -- Thermal Reference/LConn1
  Controlled Heat Flow Rate Source/LConn1 -- Temperature Sensor/LConn1 -- Battery Thermal Mass/LConn1 -- H/RConn1
  Controlled Heat Flow Rate Source/RConn1 -- P_in/RConn1

== system Ecm_2RC_battery/Subsystem4/Subsystem9/Sum ==
  Power Sum : fl_lib/Physical Signals/Functions/PS Add
      settings: SourceProductBaseCode=PW,SS,VE
  Power Sum1 : fl_lib/Physical Signals/Functions/PS Add
      settings: SourceProductBaseCode=PW,SS,VE
  I1 : PMIOPort  Side=Right
  I2 : PMIOPort  Port=2  Side=Right
  I3 : PMIOPort  Port=3  Side=Right
  O : PMIOPort  Port=4  Side=Left
  connections:
  Power Sum1/LConn1 -- I2/RConn1
  Power Sum/RConn1 -- O/RConn1
  I3/RConn1 -- Power Sum1/LConn2
  Power Sum1/RConn1 -- Power Sum/LConn2
  I1/RConn1 -- Power Sum/LConn1

== system Ecm_2RC_battery/Subsystem4/Subsystem9/Thermal Model ==
  Battery Thermal Mass : fl_lib/Thermal/Thermal Elements/Thermal Mass  mass=cell_mass kg  sp_heat=cell_Cp_heat J/kg/K  T_specify=on  T_priority=High  T=T_init K  T_nominal_specify=off  T_nominal_unit=K  T_nominal_value=1  Q_specify=off  Q_priority=None  Q=0 W  Q_nominal_specify=off  Q_nominal_unit=W  Q_nominal_value=1
      settings: SourceProductBaseCode=PW,SS,VE
  Controlled Heat Flow Rate Source : fl_lib/Thermal/Thermal Sources/Controlled Heat Flow Rate Source
      settings: SourceProductBaseCode=PW,SS,VE
  Temperature Sensor : fl_lib/Thermal/Thermal Sensors/Temperature Sensor
      settings: SourceProductBaseCode=PW,SS,VE
  Thermal Reference : fl_lib/Thermal/Thermal Elements/Thermal Reference
      settings: SourceProductBaseCode=PW,SS,VE
  Thermal Reference1 : fl_lib/Thermal/Thermal Elements/Thermal Reference
      settings: SourceProductBaseCode=PW,SS,VE
  P_in : PMIOPort  Tag=PMCPort  Side=Left
  H : PMIOPort  Tag=PMCPort  Port=2  Side=Left
  T : PMIOPort  Tag=PMCPort  Port=3  Side=Right
  connections:
  Temperature Sensor/RConn1 -- Thermal Reference1/LConn1
  Temperature Sensor/RConn2 -- T/RConn1
  Controlled Heat Flow Rate Source/RConn2 -- Thermal Reference/LConn1
  Controlled Heat Flow Rate Source/LConn1 -- Temperature Sensor/LConn1 -- Battery Thermal Mass/LConn1 -- H/RConn1
  Controlled Heat Flow Rate Source/RConn1 -- P_in/RConn1

== system Ecm_2RC_battery/Subsystem5/Subsystem/Sum ==
  Power Sum : fl_lib/Physical Signals/Functions/PS Add
      settings: SourceProductBaseCode=PW,SS,VE
  Power Sum1 : fl_lib/Physical Signals/Functions/PS Add
      settings: SourceProductBaseCode=PW,SS,VE
  I1 : PMIOPort  Side=Right
  I2 : PMIOPort  Port=2  Side=Right
  I3 : PMIOPort  Port=3  Side=Right
  O : PMIOPort  Port=4  Side=Left
  connections:
  Power Sum1/LConn1 -- I2/RConn1
  Power Sum/RConn1 -- O/RConn1
  I3/RConn1 -- Power Sum1/LConn2
  Power Sum1/RConn1 -- Power Sum/LConn2
  I1/RConn1 -- Power Sum/LConn1

== system Ecm_2RC_battery/Subsystem5/Subsystem/Thermal Model ==
  Battery Thermal Mass : fl_lib/Thermal/Thermal Elements/Thermal Mass  mass=cell_mass kg  sp_heat=cell_Cp_heat J/kg/K  T_specify=on  T_priority=High  T=T_init K  T_nominal_specify=off  T_nominal_unit=K  T_nominal_value=1  Q_specify=off  Q_priority=None  Q=0 W  Q_nominal_specify=off  Q_nominal_unit=W  Q_nominal_value=1
      settings: SourceProductBaseCode=PW,SS,VE
  Controlled Heat Flow Rate Source : fl_lib/Thermal/Thermal Sources/Controlled Heat Flow Rate Source
      settings: SourceProductBaseCode=PW,SS,VE
  Temperature Sensor : fl_lib/Thermal/Thermal Sensors/Temperature Sensor
      settings: SourceProductBaseCode=PW,SS,VE
  Thermal Reference : fl_lib/Thermal/Thermal Elements/Thermal Reference
      settings: SourceProductBaseCode=PW,SS,VE
  Thermal Reference1 : fl_lib/Thermal/Thermal Elements/Thermal Reference
      settings: SourceProductBaseCode=PW,SS,VE
  P_in : PMIOPort  Tag=PMCPort  Side=Left
  H : PMIOPort  Tag=PMCPort  Port=2  Side=Left
  T : PMIOPort  Tag=PMCPort  Port=3  Side=Right
  connections:
  Temperature Sensor/RConn1 -- Thermal Reference1/LConn1
  Temperature Sensor/RConn2 -- T/RConn1
  Controlled Heat Flow Rate Source/RConn2 -- Thermal Reference/LConn1
  Controlled Heat Flow Rate Source/LConn1 -- Temperature Sensor/LConn1 -- Battery Thermal Mass/LConn1 -- H/RConn1
  Controlled Heat Flow Rate Source/RConn1 -- P_in/RConn1

== system Ecm_2RC_battery/Subsystem5/Subsystem1/Sum ==
  Power Sum : fl_lib/Physical Signals/Functions/PS Add
      settings: SourceProductBaseCode=PW,SS,VE
  Power Sum1 : fl_lib/Physical Signals/Functions/PS Add
      settings: SourceProductBaseCode=PW,SS,VE
  I1 : PMIOPort  Side=Right
  I2 : PMIOPort  Port=2  Side=Right
  I3 : PMIOPort  Port=3  Side=Right
  O : PMIOPort  Port=4  Side=Left
  connections:
  Power Sum1/LConn1 -- I2/RConn1
  Power Sum/RConn1 -- O/RConn1
  I3/RConn1 -- Power Sum1/LConn2
  Power Sum1/RConn1 -- Power Sum/LConn2
  I1/RConn1 -- Power Sum/LConn1

== system Ecm_2RC_battery/Subsystem5/Subsystem1/Thermal Model ==
  Battery Thermal Mass : fl_lib/Thermal/Thermal Elements/Thermal Mass  mass=cell_mass kg  sp_heat=cell_Cp_heat J/kg/K  T_specify=on  T_priority=High  T=T_init K  T_nominal_specify=off  T_nominal_unit=K  T_nominal_value=1  Q_specify=off  Q_priority=None  Q=0 W  Q_nominal_specify=off  Q_nominal_unit=W  Q_nominal_value=1
      settings: SourceProductBaseCode=PW,SS,VE
  Controlled Heat Flow Rate Source : fl_lib/Thermal/Thermal Sources/Controlled Heat Flow Rate Source
      settings: SourceProductBaseCode=PW,SS,VE
  Temperature Sensor : fl_lib/Thermal/Thermal Sensors/Temperature Sensor
      settings: SourceProductBaseCode=PW,SS,VE
  Thermal Reference : fl_lib/Thermal/Thermal Elements/Thermal Reference
      settings: SourceProductBaseCode=PW,SS,VE
  Thermal Reference1 : fl_lib/Thermal/Thermal Elements/Thermal Reference
      settings: SourceProductBaseCode=PW,SS,VE
  P_in : PMIOPort  Tag=PMCPort  Side=Left
  H : PMIOPort  Tag=PMCPort  Port=2  Side=Left
  T : PMIOPort  Tag=PMCPort  Port=3  Side=Right
  connections:
  Temperature Sensor/RConn1 -- Thermal Reference1/LConn1
  Temperature Sensor/RConn2 -- T/RConn1
  Controlled Heat Flow Rate Source/RConn2 -- Thermal Reference/LConn1
  Controlled Heat Flow Rate Source/LConn1 -- Temperature Sensor/LConn1 -- Battery Thermal Mass/LConn1 -- H/RConn1
  Controlled Heat Flow Rate Source/RConn1 -- P_in/RConn1

== system Ecm_2RC_battery/Subsystem5/Subsystem2/Sum ==
  Power Sum : fl_lib/Physical Signals/Functions/PS Add
      settings: SourceProductBaseCode=PW,SS,VE
  Power Sum1 : fl_lib/Physical Signals/Functions/PS Add
      settings: SourceProductBaseCode=PW,SS,VE
  I1 : PMIOPort  Side=Right
  I2 : PMIOPort  Port=2  Side=Right
  I3 : PMIOPort  Port=3  Side=Right
  O : PMIOPort  Port=4  Side=Left
  connections:
  Power Sum1/LConn1 -- I2/RConn1
  Power Sum/RConn1 -- O/RConn1
  I3/RConn1 -- Power Sum1/LConn2
  Power Sum1/RConn1 -- Power Sum/LConn2
  I1/RConn1 -- Power Sum/LConn1

== system Ecm_2RC_battery/Subsystem5/Subsystem2/Thermal Model ==
  Battery Thermal Mass : fl_lib/Thermal/Thermal Elements/Thermal Mass  mass=cell_mass kg  sp_heat=cell_Cp_heat J/kg/K  T_specify=on  T_priority=High  T=T_init K  T_nominal_specify=off  T_nominal_unit=K  T_nominal_value=1  Q_specify=off  Q_priority=None  Q=0 W  Q_nominal_specify=off  Q_nominal_unit=W  Q_nominal_value=1
      settings: SourceProductBaseCode=PW,SS,VE
  Controlled Heat Flow Rate Source : fl_lib/Thermal/Thermal Sources/Controlled Heat Flow Rate Source
      settings: SourceProductBaseCode=PW,SS,VE
  Temperature Sensor : fl_lib/Thermal/Thermal Sensors/Temperature Sensor
      settings: SourceProductBaseCode=PW,SS,VE
  Thermal Reference : fl_lib/Thermal/Thermal Elements/Thermal Reference
      settings: SourceProductBaseCode=PW,SS,VE
  Thermal Reference1 : fl_lib/Thermal/Thermal Elements/Thermal Reference
      settings: SourceProductBaseCode=PW,SS,VE
  P_in : PMIOPort  Tag=PMCPort  Side=Left
  H : PMIOPort  Tag=PMCPort  Port=2  Side=Left
  T : PMIOPort  Tag=PMCPort  Port=3  Side=Right
  connections:
  Temperature Sensor/RConn1 -- Thermal Reference1/LConn1
  Temperature Sensor/RConn2 -- T/RConn1
  Controlled Heat Flow Rate Source/RConn2 -- Thermal Reference/LConn1
  Controlled Heat Flow Rate Source/LConn1 -- Temperature Sensor/LConn1 -- Battery Thermal Mass/LConn1 -- H/RConn1
  Controlled Heat Flow Rate Source/RConn1 -- P_in/RConn1

== system Ecm_2RC_battery/Subsystem5/Subsystem3/Sum ==
  Power Sum : fl_lib/Physical Signals/Functions/PS Add
      settings: SourceProductBaseCode=PW,SS,VE
  Power Sum1 : fl_lib/Physical Signals/Functions/PS Add
      settings: SourceProductBaseCode=PW,SS,VE
  I1 : PMIOPort  Side=Right
  I2 : PMIOPort  Port=2  Side=Right
  I3 : PMIOPort  Port=3  Side=Right
  O : PMIOPort  Port=4  Side=Left
  connections:
  Power Sum1/LConn1 -- I2/RConn1
  Power Sum/RConn1 -- O/RConn1
  I3/RConn1 -- Power Sum1/LConn2
  Power Sum1/RConn1 -- Power Sum/LConn2
  I1/RConn1 -- Power Sum/LConn1

== system Ecm_2RC_battery/Subsystem5/Subsystem3/Thermal Model ==
  Battery Thermal Mass : fl_lib/Thermal/Thermal Elements/Thermal Mass  mass=cell_mass kg  sp_heat=cell_Cp_heat J/kg/K  T_specify=on  T_priority=High  T=T_init K  T_nominal_specify=off  T_nominal_unit=K  T_nominal_value=1  Q_specify=off  Q_priority=None  Q=0 W  Q_nominal_specify=off  Q_nominal_unit=W  Q_nominal_value=1
      settings: SourceProductBaseCode=PW,SS,VE
  Controlled Heat Flow Rate Source : fl_lib/Thermal/Thermal Sources/Controlled Heat Flow Rate Source
      settings: SourceProductBaseCode=PW,SS,VE
  Temperature Sensor : fl_lib/Thermal/Thermal Sensors/Temperature Sensor
      settings: SourceProductBaseCode=PW,SS,VE
  Thermal Reference : fl_lib/Thermal/Thermal Elements/Thermal Reference
      settings: SourceProductBaseCode=PW,SS,VE
  Thermal Reference1 : fl_lib/Thermal/Thermal Elements/Thermal Reference
      settings: SourceProductBaseCode=PW,SS,VE
  P_in : PMIOPort  Tag=PMCPort  Side=Left
  H : PMIOPort  Tag=PMCPort  Port=2  Side=Left
  T : PMIOPort  Tag=PMCPort  Port=3  Side=Right
  connections:
  Temperature Sensor/RConn1 -- Thermal Reference1/LConn1
  Temperature Sensor/RConn2 -- T/RConn1
  Controlled Heat Flow Rate Source/RConn2 -- Thermal Reference/LConn1
  Controlled Heat Flow Rate Source/LConn1 -- Temperature Sensor/LConn1 -- Battery Thermal Mass/LConn1 -- H/RConn1
  Controlled Heat Flow Rate Source/RConn1 -- P_in/RConn1

== system Ecm_2RC_battery/Subsystem5/Subsystem4/Sum ==
  Power Sum : fl_lib/Physical Signals/Functions/PS Add
      settings: SourceProductBaseCode=PW,SS,VE
  Power Sum1 : fl_lib/Physical Signals/Functions/PS Add
      settings: SourceProductBaseCode=PW,SS,VE
  I1 : PMIOPort  Side=Right
  I2 : PMIOPort  Port=2  Side=Right
  I3 : PMIOPort  Port=3  Side=Right
  O : PMIOPort  Port=4  Side=Left
  connections:
  Power Sum1/LConn1 -- I2/RConn1
  Power Sum/RConn1 -- O/RConn1
  I3/RConn1 -- Power Sum1/LConn2
  Power Sum1/RConn1 -- Power Sum/LConn2
  I1/RConn1 -- Power Sum/LConn1

== system Ecm_2RC_battery/Subsystem5/Subsystem4/Thermal Model ==
  Battery Thermal Mass : fl_lib/Thermal/Thermal Elements/Thermal Mass  mass=cell_mass kg  sp_heat=cell_Cp_heat J/kg/K  T_specify=on  T_priority=High  T=T_init K  T_nominal_specify=off  T_nominal_unit=K  T_nominal_value=1  Q_specify=off  Q_priority=None  Q=0 W  Q_nominal_specify=off  Q_nominal_unit=W  Q_nominal_value=1
      settings: SourceProductBaseCode=PW,SS,VE
  Controlled Heat Flow Rate Source : fl_lib/Thermal/Thermal Sources/Controlled Heat Flow Rate Source
      settings: SourceProductBaseCode=PW,SS,VE
  Temperature Sensor : fl_lib/Thermal/Thermal Sensors/Temperature Sensor
      settings: SourceProductBaseCode=PW,SS,VE
  Thermal Reference : fl_lib/Thermal/Thermal Elements/Thermal Reference
      settings: SourceProductBaseCode=PW,SS,VE
  Thermal Reference1 : fl_lib/Thermal/Thermal Elements/Thermal Reference
      settings: SourceProductBaseCode=PW,SS,VE
  P_in : PMIOPort  Tag=PMCPort  Side=Left
  H : PMIOPort  Tag=PMCPort  Port=2  Side=Left
  T : PMIOPort  Tag=PMCPort  Port=3  Side=Right
  connections:
  Temperature Sensor/RConn1 -- Thermal Reference1/LConn1
  Temperature Sensor/RConn2 -- T/RConn1
  Controlled Heat Flow Rate Source/RConn2 -- Thermal Reference/LConn1
  Controlled Heat Flow Rate Source/LConn1 -- Temperature Sensor/LConn1 -- Battery Thermal Mass/LConn1 -- H/RConn1
  Controlled Heat Flow Rate Source/RConn1 -- P_in/RConn1

== system Ecm_2RC_battery/Subsystem5/Subsystem5/Sum ==
  Power Sum : fl_lib/Physical Signals/Functions/PS Add
      settings: SourceProductBaseCode=PW,SS,VE
  Power Sum1 : fl_lib/Physical Signals/Functions/PS Add
      settings: SourceProductBaseCode=PW,SS,VE
  I1 : PMIOPort  Side=Right
  I2 : PMIOPort  Port=2  Side=Right
  I3 : PMIOPort  Port=3  Side=Right
  O : PMIOPort  Port=4  Side=Left
  connections:
  Power Sum1/LConn1 -- I2/RConn1
  Power Sum/RConn1 -- O/RConn1
  I3/RConn1 -- Power Sum1/LConn2
  Power Sum1/RConn1 -- Power Sum/LConn2
  I1/RConn1 -- Power Sum/LConn1

== system Ecm_2RC_battery/Subsystem5/Subsystem5/Thermal Model ==
  Battery Thermal Mass : fl_lib/Thermal/Thermal Elements/Thermal Mass  mass=cell_mass kg  sp_heat=cell_Cp_heat J/kg/K  T_specify=on  T_priority=High  T=T_init K  T_nominal_specify=off  T_nominal_unit=K  T_nominal_value=1  Q_specify=off  Q_priority=None  Q=0 W  Q_nominal_specify=off  Q_nominal_unit=W  Q_nominal_value=1
      settings: SourceProductBaseCode=PW,SS,VE
  Controlled Heat Flow Rate Source : fl_lib/Thermal/Thermal Sources/Controlled Heat Flow Rate Source
      settings: SourceProductBaseCode=PW,SS,VE
  Temperature Sensor : fl_lib/Thermal/Thermal Sensors/Temperature Sensor
      settings: SourceProductBaseCode=PW,SS,VE
  Thermal Reference : fl_lib/Thermal/Thermal Elements/Thermal Reference
      settings: SourceProductBaseCode=PW,SS,VE
  Thermal Reference1 : fl_lib/Thermal/Thermal Elements/Thermal Reference
      settings: SourceProductBaseCode=PW,SS,VE
  P_in : PMIOPort  Tag=PMCPort  Side=Left
  H : PMIOPort  Tag=PMCPort  Port=2  Side=Left
  T : PMIOPort  Tag=PMCPort  Port=3  Side=Right
  connections:
  Temperature Sensor/RConn1 -- Thermal Reference1/LConn1
  Temperature Sensor/RConn2 -- T/RConn1
  Controlled Heat Flow Rate Source/RConn2 -- Thermal Reference/LConn1
  Controlled Heat Flow Rate Source/LConn1 -- Temperature Sensor/LConn1 -- Battery Thermal Mass/LConn1 -- H/RConn1
  Controlled Heat Flow Rate Source/RConn1 -- P_in/RConn1

== system Ecm_2RC_battery/Subsystem5/Subsystem6/Sum ==
  Power Sum : fl_lib/Physical Signals/Functions/PS Add
      settings: SourceProductBaseCode=PW,SS,VE
  Power Sum1 : fl_lib/Physical Signals/Functions/PS Add
      settings: SourceProductBaseCode=PW,SS,VE
  I1 : PMIOPort  Side=Right
  I2 : PMIOPort  Port=2  Side=Right
  I3 : PMIOPort  Port=3  Side=Right
  O : PMIOPort  Port=4  Side=Left
  connections:
  Power Sum1/LConn1 -- I2/RConn1
  Power Sum/RConn1 -- O/RConn1
  I3/RConn1 -- Power Sum1/LConn2
  Power Sum1/RConn1 -- Power Sum/LConn2
  I1/RConn1 -- Power Sum/LConn1

== system Ecm_2RC_battery/Subsystem5/Subsystem6/Thermal Model ==
  Battery Thermal Mass : fl_lib/Thermal/Thermal Elements/Thermal Mass  mass=cell_mass kg  sp_heat=cell_Cp_heat J/kg/K  T_specify=on  T_priority=High  T=T_init K  T_nominal_specify=off  T_nominal_unit=K  T_nominal_value=1  Q_specify=off  Q_priority=None  Q=0 W  Q_nominal_specify=off  Q_nominal_unit=W  Q_nominal_value=1
      settings: SourceProductBaseCode=PW,SS,VE
  Controlled Heat Flow Rate Source : fl_lib/Thermal/Thermal Sources/Controlled Heat Flow Rate Source
      settings: SourceProductBaseCode=PW,SS,VE
  Temperature Sensor : fl_lib/Thermal/Thermal Sensors/Temperature Sensor
      settings: SourceProductBaseCode=PW,SS,VE
  Thermal Reference : fl_lib/Thermal/Thermal Elements/Thermal Reference
      settings: SourceProductBaseCode=PW,SS,VE
  Thermal Reference1 : fl_lib/Thermal/Thermal Elements/Thermal Reference
      settings: SourceProductBaseCode=PW,SS,VE
  P_in : PMIOPort  Tag=PMCPort  Side=Left
  H : PMIOPort  Tag=PMCPort  Port=2  Side=Left
  T : PMIOPort  Tag=PMCPort  Port=3  Side=Right
  connections:
  Temperature Sensor/RConn1 -- Thermal Reference1/LConn1
  Temperature Sensor/RConn2 -- T/RConn1
  Controlled Heat Flow Rate Source/RConn2 -- Thermal Reference/LConn1
  Controlled Heat Flow Rate Source/LConn1 -- Temperature Sensor/LConn1 -- Battery Thermal Mass/LConn1 -- H/RConn1
  Controlled Heat Flow Rate Source/RConn1 -- P_in/RConn1
